simulink model "untitled"  (Simulink 7.3)
settings: Solver=ode45  StartTime=0.0  StopTime=10.0  RelTol=1e-3
settings Model: Creator=Administrator  LastModifiedBy=Administrator

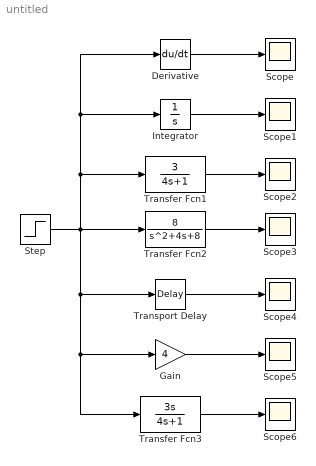
== system untitled ==
  Derivative : Derivative
  Gain : Gain  Gain=4  ParameterDataType=fixdt(1, 16)  ParameterScaling=2^0  OutDataType=fixdt(1, 16)  OutScaling=2^0
  Integrator : Integrator
  Scope{,1..6} (7 alike) : Scope
      Scope2 settings: SaveName=ScopeData2
      Scope3 settings: SaveName=ScopeData3
      Scope4 settings: SaveName=ScopeData4
      Scope5 settings: SaveName=ScopeData5
      Scope6 settings: SaveName=ScopeData6
  Step : Step  SampleTime=0
  Transfer Fcn1 : TransferFcn  Numerator=[3]  Denominator=[4 1]
  Transfer Fcn2 : TransferFcn  Numerator=[8]  Denominator=[1 4 8]
  Transfer Fcn3 : TransferFcn  Numerator=[3 0]  Denominator=[4 1]
  Transport Delay : TransportDelay
  wires:
  Step/1 -> Transfer Fcn2/1, Transfer Fcn1/1, Integrator/1, Derivative/1, Transport Delay/1, Gain/1, Transfer Fcn3/1
  Transfer Fcn3/1 -> Scope6/1
  Gain/1 -> Scope5/1
  Transport Delay/1 -> Scope4/1
  Transfer Fcn2/1 -> Scope3/1
  Transfer Fcn1/1 -> Scope2/1
  Integrator/1 -> Scope1/1
  Derivative/1 -> Scope/1
